simulink model "velo_p"  (Simulink 9.2)
settings: Solver=FixedStepDiscrete  StartTime=0.0  StopTime=10.0  RelTol=1e-3  EnableMultiTasking=on
undefined symbols (not defined in the file or in its folder): ts
libraries: arduino_io_lib x5
settings Model: Creator=hirata  LastModifiedBy=is221042
settings OptimizationCC: ExpressionDepthLimit=2147483647
settings DebuggingCC: SolverPrmCheckMsg=warning  SFExecutionAtInitializationDiag=warning
settings GRTTargetCC: CombineOutputUpdateFcns=on  GRTInterface=off

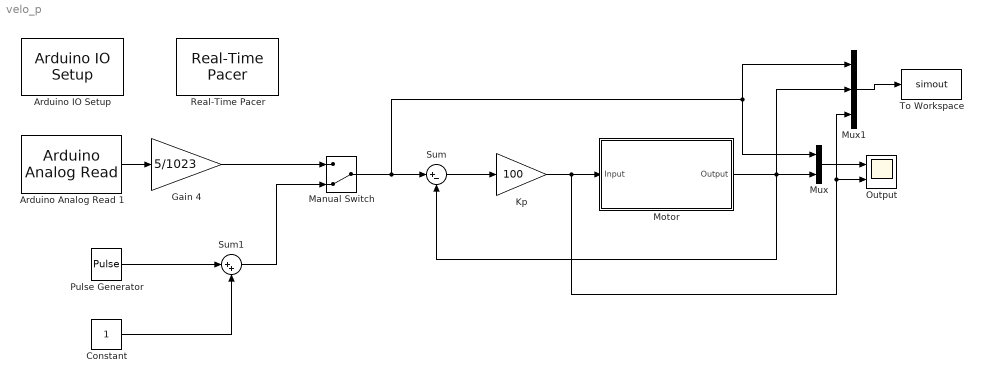
== system velo_p ==
  Arduino Analog Read 1 : arduino_io_lib/Arduino Analog Read  arduinoVar=Temporary arduino variable: Arduino1  arduinoPin=1  T=ts
  Arduino IO Setup : arduino_io_lib/Arduino IO Setup  Priority=3  arduinoVar=Temporary arduino variable: Arduino1  workspaceVarName=a  comPort=/dev/ttyACM0
  Constant : Constant
  Gain 4 : Gain  Gain=5/1023
  Kp : Gain  Gain=100
  Manual Switch : ManualSwitch  CurrentSetting=0
  Motor : Subsystem
  Mux : Mux  Inputs=2
  Mux1 : Mux  Inputs=3
  Output : Scope  NumInputPorts=2
  Pulse Generator : DiscretePulseGenerator  Amplitude=0.5  Period=4/ts  PulseWidth=2/ts  SampleTime=ts
  Real-Time Pacer : arduino_io_lib/Real-Time Pacer  simTimePerRealTime=1
  Sum : Sum  Inputs=|+-
  Sum1 : Sum  Inputs=|++
  To Workspace : ToWorkspace  VariableName=simout  SaveFormat=Timeseries  SampleTime=-1
  wires:
  Arduino Analog Read 1/1 -> Gain 4/1
  Gain 4/1 -> Manual Switch/1
  Constant/1 -> Sum1/2
  Pulse Generator/1 -> Sum1/1
  Sum1/1 -> Manual Switch/2
  Manual Switch/1 -> Sum/1, Mux1/1, Mux/1
  Sum/1 -> Kp/1
  Kp/1 -> Motor/1(Input), Mux1/3, Output/2
  Mux/1 -> Output/1
  Motor/1(Output) -> Sum/2, Mux/2, Mux1/2
  Mux1/1 -> To Workspace/1

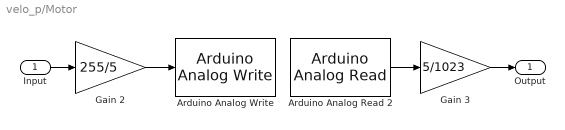
== system velo_p/Motor ==
  Input : Inport
  Arduino Analog Read 2 : arduino_io_lib/Arduino Analog Read  arduinoVar=Temporary arduino variable: Arduino1  arduinoPin=0  T=ts
  Arduino Analog Write : arduino_io_lib/Arduino Analog Write  arduinoVar=Temporary arduino variable: Arduino1  arduinoPin=3  T=ts
  Gain 2 : Gain  Gain=255/5
  Gain 3 : Gain  Gain=5/1023
  Output : Outport
  wires:
  Arduino Analog Read 2/1 -> Gain 3/1
  Gain 2/1 -> Arduino Analog Write/1
  Input/1 -> Gain 2/1
  Gain 3/1 -> Output/1
